simulink model "Trasmisor_lab"  (R2024b)
settings: Solver=VariableStepAuto  StartTime=0.0  StopTime=1  RelTol=1e-3
undefined symbols (not defined in the file or in its folder): Ts
libraries: dspsrcs4 x6, commanabbnd3 x2
settings Model: Creator=river  LastModifiedBy=RomaW11

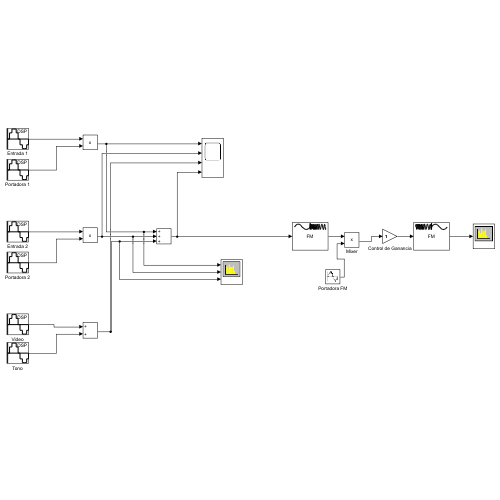
[thumbnail: Simulink's stored preview of the top-level diagram]
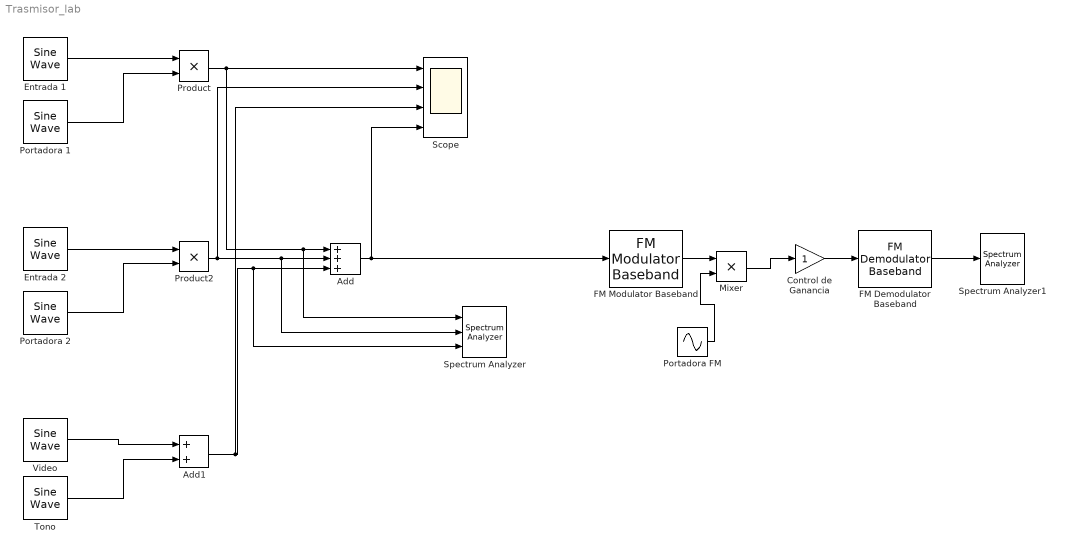
== system Trasmisor_lab ==
  Add : Sum  Inputs=+++
  Add1 : Sum
  Control de Ganancia : Gain
  Entrada 1 : dspsrcs4/Sine Wave  Amplitude=1  Frequency=15e3  Phase=0  SampleMode=Discrete  OutComplex=Real  CompMethod=Trigonometric fcn  TableSize=Speed  SampleTime=Ts*0.5  SamplesPerFrame=1  ResetState=Restart at time zero  OutputFrames=off  dataType=double  wordLen=16  udDataType=sfix(16)  fracBitsMode=Best precision  numFracBits=15  OutDataTypeStr=double  LastOutDataTypeStr=double
  Entrada 2 : dspsrcs4/Sine Wave  Amplitude=1  Frequency=15e3  Phase=0  SampleMode=Discrete  OutComplex=Real  CompMethod=Trigonometric fcn  TableSize=Speed  SampleTime=Ts*0.5  SamplesPerFrame=1  ResetState=Restart at time zero  OutputFrames=off  dataType=double  wordLen=16  udDataType=sfix(16)  fracBitsMode=Best precision  numFracBits=15  OutDataTypeStr=double  LastOutDataTypeStr=double
  "FM Demodulator Baseband " : commanabbnd3/FM Demodulator Baseband   FrequencyDeviation=75e3  SimulateUsing=Code generation
  FM Modulator Baseband : commanabbnd3/FM Modulator Baseband  FrequencyDeviation=75e3  SimulateUsing=Code generation
  Mixer : Product
  Portadora 1 : dspsrcs4/Sine Wave  Amplitude=1  Frequency=4.3e6  Phase=0  SampleMode=Discrete  OutComplex=Real  CompMethod=Trigonometric fcn  TableSize=Speed  SampleTime=Ts*0.5  SamplesPerFrame=1  ResetState=Restart at time zero  OutputFrames=off  dataType=double  wordLen=16  udDataType=sfix(16)  fracBitsMode=Best precision  numFracBits=15  OutDataTypeStr=double  LastOutDataTypeStr=double
  Portadora 2 : dspsrcs4/Sine Wave  Amplitude=1  Frequency=4.4e6  Phase=0  SampleMode=Discrete  OutComplex=Real  CompMethod=Trigonometric fcn  TableSize=Speed  SampleTime=Ts*0.5  SamplesPerFrame=1  ResetState=Restart at time zero  OutputFrames=off  dataType=double  wordLen=16  udDataType=sfix(16)  fracBitsMode=Best precision  numFracBits=15  OutDataTypeStr=double  LastOutDataTypeStr=double
  Portadora FM : Sin  Frequency=2*pi*2.45e9  SampleTime=Ts*0.5
  Product : Product
  Product2 : Product
  Scope : Scope  NumInputPorts=4
  Spectrum Analyzer : SpectrumAnalyzer  NumInputPorts=3  WindowPosition=[962.000000,50.000000,958.000000,1000.000000,]  ScopeFrameLocation=window  Span=5849645.520984195  StartFrequency=-2924822.7604920976  StopFrequency=2924822.7604920976  YLimits=[-256.17682941,55.10786864]  SelectedToolstripTab=spectrumAnalyzerToolstrip.spectrumTab
  Spectrum Analyzer1 : SpectrumAnalyzer  WindowPosition=[0.000000,36.000000,1536.000000,792.000000,]  ScopeFrameLocation=window  Span=5849645.520984195  StartFrequency=-2924822.7604920976  StopFrequency=2924822.7604920976  YLimits=[15.5339,53.7266]  SelectedToolstripTab=spectrumAnalyzerToolstrip.channelMeasurementsTab
  Tono : dspsrcs4/Sine Wave  Amplitude=1  Frequency=3.5e6  Phase=0  SampleMode=Discrete  OutComplex=Real  CompMethod=Trigonometric fcn  TableSize=Speed  SampleTime=Ts*0.5  SamplesPerFrame=1  ResetState=Restart at time zero  OutputFrames=off  dataType=double  wordLen=16  udDataType=sfix(16)  fracBitsMode=Best precision  numFracBits=15  OutDataTypeStr=double  LastOutDataTypeStr=double
  Video : dspsrcs4/Sine Wave  Amplitude=1  Frequency=3e6  Phase=0  SampleMode=Discrete  OutComplex=Real  CompMethod=Trigonometric fcn  TableSize=Speed  SampleTime=Ts*0.5  SamplesPerFrame=1  ResetState=Restart at time zero  OutputFrames=off  dataType=double  wordLen=16  udDataType=sfix(16)  fracBitsMode=Best precision  numFracBits=15  OutDataTypeStr=double  LastOutDataTypeStr=double
  wires:
  Product2/1 -> Scope/2, Spectrum Analyzer/2, Add/2
  Add1/1 -> Scope/3, Spectrum Analyzer/3, Add/3
  Product/1 -> Spectrum Analyzer/1, Add/1, Scope/1
  Portadora 1/1 -> Product/2
  Portadora 2/1 -> Product2/2
  Video/1 -> Add1/1
  Tono/1 -> Add1/2
  Entrada 1/1 -> Product/1
  Entrada 2/1 -> Product2/1
  Portadora FM/1 -> Mixer/2
  Control de Ganancia/1 -> "FM Demodulator Baseband "/1
  Mixer/1 -> Control de Ganancia/1
  FM Modulator Baseband/1 -> Mixer/1
  Add/1 -> FM Modulator Baseband/1, Scope/4
  "FM Demodulator Baseband "/1 -> Spectrum Analyzer1/1
